simulink model "task3"  (R2024a)
settings: Solver=ode45  StartTime=0.0  StopTime=10  FixedStep=0.01  MaxStep=0.01  RelTol=1e-3
undefined symbols (not defined in the file): A, B, C, D, K, L, x0, x0_hat
settings Model: Creator=sizgr  LastModifiedBy=sizgr

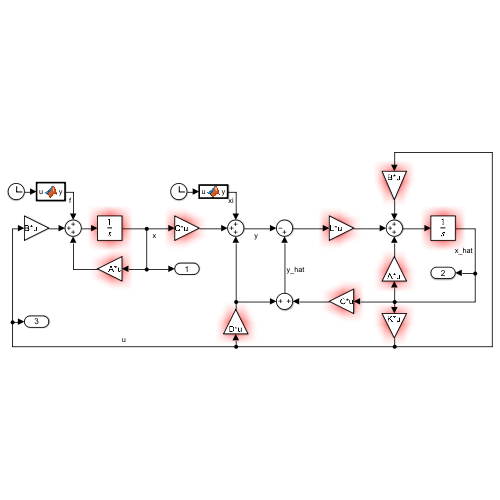
[thumbnail: Simulink's stored preview of the top-level diagram]
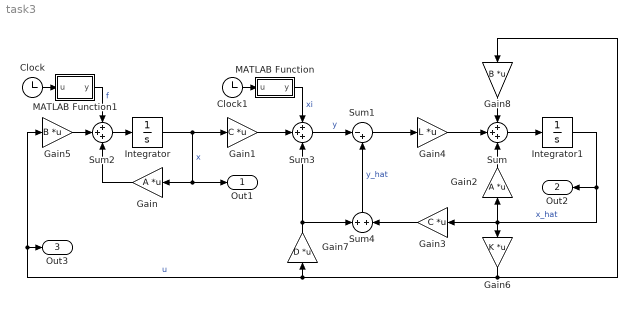
== system task3 ==
  Clock : Clock
  Clock1 : Clock
  Gain : Gain  Gain=A  Multiplication=Matrix(K*u)
  Gain1 : Gain  Gain=C  Multiplication=Matrix(K*u)
  Gain2 : Gain  Gain=A  Multiplication=Matrix(K*u)
  Gain3 : Gain  Gain=C  Multiplication=Matrix(K*u)
  Gain4 : Gain  Gain=L  Multiplication=Matrix(K*u)
  Gain5 : Gain  Gain=B  Multiplication=Matrix(K*u)
  Gain6 : Gain  Gain=K  Multiplication=Matrix(K*u)
  Gain7 : Gain  Gain=D  Multiplication=Matrix(K*u)
  Gain8 : Gain  Gain=B  Multiplication=Matrix(K*u)
  Integrator : Integrator  InitialCondition=x0
  Integrator1 : Integrator  InitialCondition=x0_hat
  MATLAB Function : MATLAB Function  TreatAsAtomicUnit=on
  MATLAB Function1 : MATLAB Function  TreatAsAtomicUnit=on
  Sum : Sum  Inputs=+++
  Sum1 : Sum  Inputs=|-+
  Sum2 : Sum  Inputs=+++
  Sum3 : Sum  Inputs=+++
  Sum4 : Sum  Inputs=+|+
  Out1 : Outport
  Out2 : Outport  Port=2
  Out3 : Outport  Port=3
  wires:
  Integrator/1 -> Out1/1, Gain/1, Gain1/1  "x"
  Gain/1 -> Sum2/3
  Integrator1/1 -> Out2/1, Gain3/1, Gain6/1, Gain2/1  "x_hat"
  Sum/1 -> Integrator1/1
  Sum1/1 -> Gain4/1
  Sum2/1 -> Integrator/1
  MATLAB Function1/1(y) -> Sum2/1  "f"
  Sum3/1 -> Sum1/1  "y"
  Clock/1 -> MATLAB Function1/1(u)
  Gain5/1 -> Sum2/2
  Clock1/1 -> MATLAB Function/1(u)
  Gain6/1 -> Gain7/1, Out3/1, Gain5/1, Gain8/1  "u"
  Gain1/1 -> Sum3/2
  MATLAB Function/1(y) -> Sum3/1  "xi"
  Gain7/1 -> Sum3/3, Sum4/1
  Gain4/1 -> Sum/2
  Gain2/1 -> Sum/3
  Gain8/1 -> Sum/1
  Sum4/1 -> Sum1/2  "y_hat"
  Gain3/1 -> Sum4/2

== matlab function task3/MATLAB Function ==
  data: u input; y output
function y = fcn(u)

y = [0.2*sin(2*u); 0.2*sin(5*u)];

== matlab function task3/MATLAB Function1 ==
  data: u input; y output
function y = fcn(u)

y = [0.1*cos(0.5*u); 0.1*cos(u); 0.1*cos(0.5*u); 0.1*cos(u)];
